simulink model "DoubleTankSim_FeedbackLin"  (R2025b)
settings: Solver=ode5  StartTime=0.0  StopTime=1500  FixedStep=Ts  RelTol=1e-3  EnableMultiTasking=on
values from neighbouring files (symbols this model uses):
  a_1 = 0.15025    [LabC.m]
  a_2 = 0.15615    [LabC.m]
  At = 33    [LabC.m]
  g = 981    [LabC.m]
  h_0 = 3.2    [LabC.m]
  h_1 = [2.5 3 3.5 4 4.5 5 5.5 6 6.5 7 7.5 8 8.5 9 9.5 10 10.5 11 11.5 12 12.5 13 13.5 14.5 15]    [LabC.m]
  h_2 = [3 3.5 4 4.5 5 5.5 6 6.5 7 7.5 8 8.5 9 9.5 10 10.5 11 11.5 12 12.5 13 13.5 14 14.5 15]    [LabC.m]
  h_2_V = [0.75 1.03 1.47 1.85 2.22 2.61 2.93 3.35 3.72 4.09 4.49 4.88 5.21 5.62 6.00 6.33 6.75  7.13 7.50 7.94 8.29 8.65 9.03 9.38 9.77]    [LabC.m]
  height_limit = 15.5    [LabC.m]
  height_safe = 0.9 * height_limit    (= 13.95)    [LabC.m]
  Kd = 12 * zeta * omega_n    (= 0.64)    [LabC.m]
  Ki = 10 * zeta * omega_n^3    (= 0.00151703703704)    [LabC.m]
  Kp = omega_n^2 * (1 + 20*zeta^2)    (= 0.0597333333333)    [LabC.m]
  N = 1    [LabC.m]
  omega_n = 4/(zeta*T_s_cl)    (= 0.0533333333333)    [LabC.m]
  Q = [variance 0 0 ... (first row only)    [LabC.m]
  R = 1    [LabC.m]
  R_2d = diag([1, 1])    [LabC.m]
  tau = T_s_cl/2    (= 37.5)    [LabC.m]
  Ts = 0.02    [LabC.m]
undefined symbols (not defined in the file or in its folder): h_1_V, National_Instruments, PCIe
libraries: sldrtlib x2, simulink x2, slpidlib x2
settings Model: Creator=William  LastModifiedBy=William
settings SolverCC: AutoInsertRateTranBlk=on

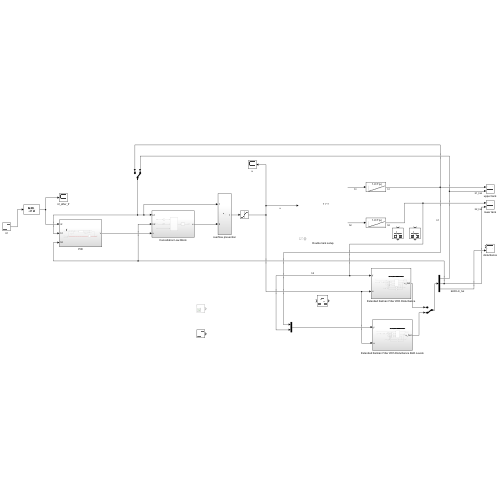
[thumbnail: Simulink's stored preview of the top-level diagram]
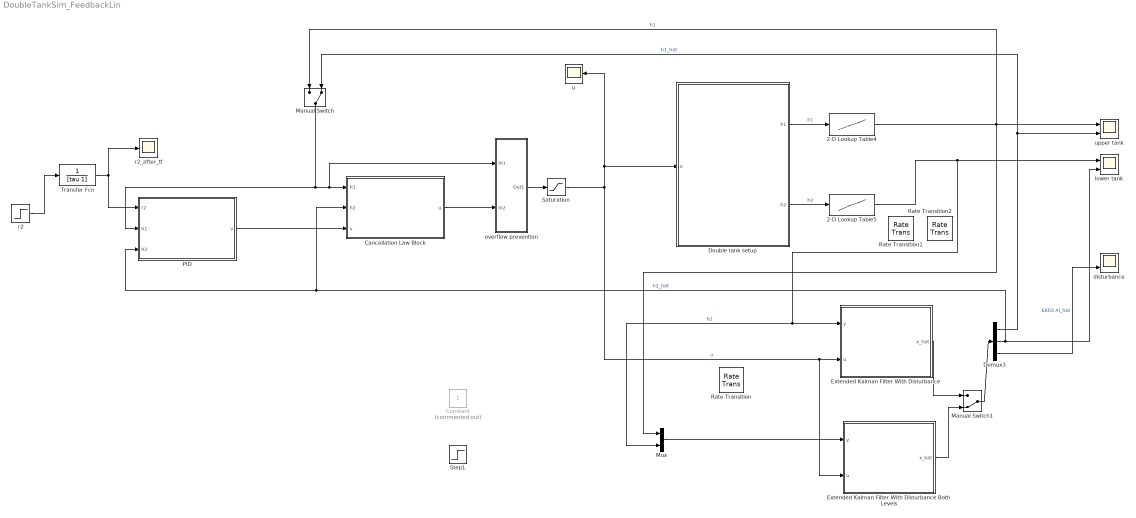
== system DoubleTankSim_FeedbackLin ==
  2-D Lookup Table4 : Lookup_n-D  NumberOfTableDimensions=1  BreakpointsForDimension1=x  BreakpointsForDimension2=[1:3]  Table=y  RndMeth=Simplest  mask{x=h_1_V, y=h_1}
      mask prompts: x "Values on x-axis"; y "Values on y-axis"
  2-D Lookup Table5 : Lookup_n-D  NumberOfTableDimensions=1  BreakpointsForDimension1=x  BreakpointsForDimension2=[1:3]  Table=y  RndMeth=Simplest  mask{x=h_2_V, y=h_2}
      mask prompts: x "Values on x-axis"; y "Values on y-axis"
  Cancellation Law Block : Subsystem
  Constant : Constant  Commented=on
  Demux3 : Demux  Outputs=3
  Double tank setup : Subsystem  AncestorBlock=R7014E_lib/Double tank setup  StopFcn=|  mask(Realtime interface for the tank process){ts=0.02, h1_ch=0, h2_ch=1, u_ch=0}
      | chn =get_param(gcb,'u_ch');                          
      | s = daq.createSession('ni');                         
      | channel = ['ao',chn];                                
      | s.addAnalogOutputChannel('Dev1', channel, 'Voltage');
      | x = zeros(5,1);                                      
      | s.queueOutputData(x);                                
      | lh = s.addlistener('DataRequired', ...               
      | @(src,event) src.queueOutputData(x));                
      | s.startBackground();                                 
      | s.wait();                                            
      | s.stop();                                            
      | delete(lh);                                          
      | clear chn;                                           
      | clear s;                                             
      | clear channel;                                       
      | clear lh;                                            
      | clear x;
      mask prompts: ts "Sample time"; h1_ch "A/D Channel for upper tank"; h2_ch "A/D Channel for lower tank"; u_ch "D/A Channel for pump"
      mask help:
      | This block represents the physical interface from the computer to the tank process.
      |
      | The input u is the voltage that is provided for the pump, the output h1 is the measured level in the upper tank in [V] and the output h2 is the
      | measured level in the lower tank in [V].
      |
      | You need to provide the sample rate at which the voltage to the pump is updated and the level measurements are sampled. The sample rate should not be less than 0.02 seconds.
      mask Display:
      | x=363;
      | y=381;
      | image(imread('tank_icon.jpg'));
      | text(250/x,309/y,'Sensor');
      | text(260/x,169/y,'Sensor');
      | text(335/x,289/y,'A');
      | text(351/x,283/y,'D');
      | text(335/x,100/y,'A');
      | text(351/x,95/y,'D');
      | text(22/x,187/y,'A');
      | text(5/x,195/y,'D');
      | text(225/x,278/y,'h_1','texmode','on');
      | text(225/x,146/y,'h_2','texmode','on');
      | text(300/x,270/y,sprintf('AI-%d',h1_ch));
      | text(300/x,80/y,sprintf('AI-%d',h2_ch));
      | text(40/x,173/y,sprintf('AO-%d',u_ch));
  Extended Kalman Filter With Disturbance : Subsystem
  Extended Kalman Filter With Disturbance Both Levels : Subsystem
  Manual Switch : ManualSwitch  CurrentSetting=0
  Manual Switch1 : ManualSwitch  CurrentSetting=0
  Mux : Mux  Inputs=2
  PID : Subsystem
  Rate Transition : RateTransition  OutPortSampleTime=Ts
  Rate Transition1 : RateTransition  OutPortSampleTime=Ts
  Rate Transition2 : RateTransition  OutPortSampleTime=Ts
  Saturation : Saturate  UpperLimit=10  LowerLimit=0
  Step1 : Step  Time=750  Before=1  After=1.25  SampleTime=0
  Transfer Fcn : TransferFcn  Denominator=[tau 1]
  disturbance : Scope  NumInputPorts=2
      settings: ActiveDisplayYMinimum=-0.015496470014474377  ActiveDisplayYMaximum=0.13931374108372324  DataLoggingVariableName=ScopeData2
  lower tank : Scope  NumInputPorts=2
      settings: ActiveDisplayYMinimum=-1.8057811743118082  ActiveDisplayYMaximum=15.777371038796296
  overflow prevention : Subsystem
  r2 : Step  Time=500  Before=8  After=13.95  SampleTime=0
  r2_after_tf : Scope
      settings: ActiveDisplayYMinimum=-1.7437499999996442  ActiveDisplayYMaximum=15.693749999996802  DataLoggingVariableName=ScopeData4
  u : Scope
      settings: ActiveDisplayYMinimum=-1.2499999999999998  ActiveDisplayYMaximum=11.25  DataLoggingVariableName=ScopeData3
  upper tank : Scope  NumInputPorts=2
      settings: ActiveDisplayYMinimum=-1.9029859274386325  ActiveDisplayYMaximum=16.774636482282123
  wires:
  overflow prevention/1(Out1) -> Saturation/1
  Mux/1 -> Extended Kalman Filter With Disturbance Both Levels/1(y)
  Extended Kalman Filter With Disturbance Both Levels/1(x_hat) -> Manual Switch1/2
  Manual Switch1/1 -> Demux3/1
  PID/1(v) -> Cancellation Law Block/3(v)
  r2/1 -> Transfer Fcn/1
  Manual Switch/1 -> PID/2(h1), overflow prevention/1(In1), Cancellation Law Block/1(h1)
  Transfer Fcn/1 -> r2_after_tf/1, PID/1(r2)
  Extended Kalman Filter With Disturbance/1(x_hat) -> Manual Switch1/1
  Demux3/3 -> disturbance/2  "EKFD Al_hat"
  Cancellation Law Block/1(u) -> overflow prevention/2(In2)
  Saturation/1 -> Extended Kalman Filter With Disturbance Both Levels/2(u), Extended Kalman Filter With Disturbance/2(u), u/1, Double tank setup/1(u)  "u"
  Demux3/1 -> upper tank/2, Manual Switch/2  "h1_hat"
  Double tank setup/1(h1) -> 2-D Lookup Table4/1  "h1"
  Demux3/2 -> PID/3(h2), Cancellation Law Block/2(h2), lower tank/2  "h2_hat"
  Double tank setup/2(h2) -> 2-D Lookup Table5/1  "h2"
  2-D Lookup Table4/1 -> Mux/1, upper tank/1, Manual Switch/1  "h1"
  2-D Lookup Table5/1 -> Mux/2, Extended Kalman Filter With Disturbance/1(y), lower tank/1  "h2"

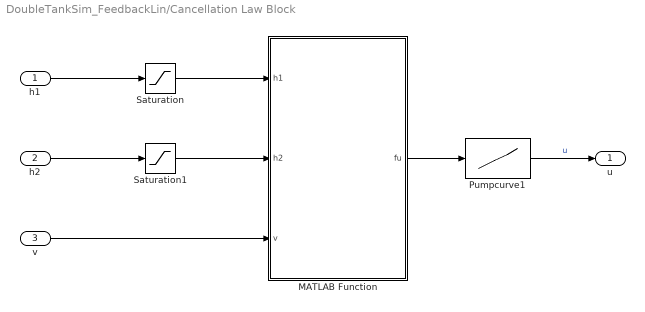
== system DoubleTankSim_FeedbackLin/Cancellation Law Block ==
  h1 : Inport
  h2 : Inport  Port=2
  v : Inport  Port=3
  MATLAB Function : MATLAB Function  TreatAsAtomicUnit=on
  Pumpcurve1 : Lookup_n-D  NumberOfTableDimensions=1  BreakpointsForDimension1=x  BreakpointsForDimension2=[1:3]  Table=y  RndMeth=Simplest  mask{x=[16.47,20.75,24.52,27.63,30.06,32.49,34.80,40.28,48.24,52.43], y=[0.5,1,1.5,2,2.5,3,3.5,5,8,10]}
      mask prompts: x "Values on x-axis"; y "Values on y-axis"
  Saturation : Saturate  UpperLimit=15.5  LowerLimit=0.001
  Saturation1 : Saturate  UpperLimit=15.5  LowerLimit=0.001
  u : Outport
  wires:
  MATLAB Function/1(fu) -> Pumpcurve1/1
  h1/1 -> Saturation/1
  h2/1 -> Saturation1/1
  Pumpcurve1/1 -> u/1  "u"
  v/1 -> MATLAB Function/3(v)
  Saturation/1 -> MATLAB Function/1(h1)
  Saturation1/1 -> MATLAB Function/2(h2)

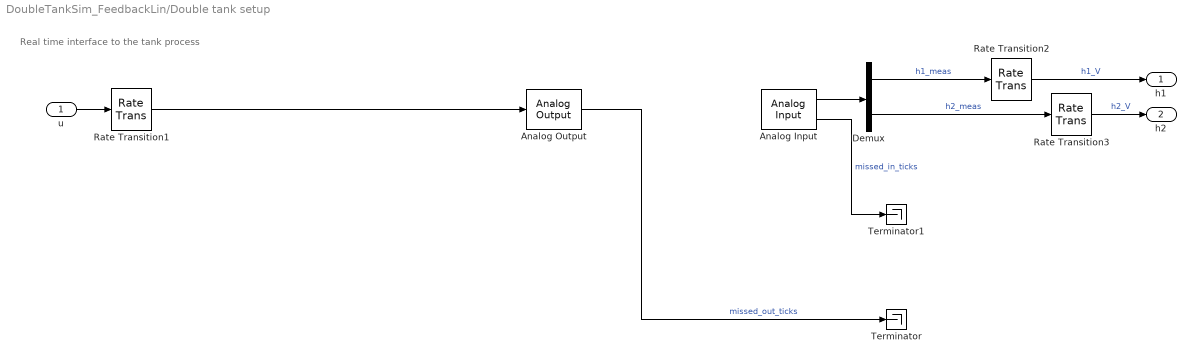
== system DoubleTankSim_FeedbackLin/Double tank setup ==
  note: Real time interface to the tank process
  u : Inport
  Analog Input : sldrtlib/Analog Input  SampleTime=ts  MaxMissedTicks=500000000  ShowMissedTicks=on  YieldWhenWaiting=off  DrvName=National_Instruments/PCIe-6321  DrvAddress=4294967295  DrvOptions=[0 0 0 0 0 0 0]  Channels=[h1_ch+1,h2_ch+1]  RangeMode=1  VoltRange=1  DataType=1
      settings: AttributesFormatString=National Instruments\nPCIe-6321 [auto]
  Analog Output : sldrtlib/Analog Output  SampleTime=ts  MaxMissedTicks=500000000  ShowMissedTicks=on  YieldWhenWaiting=off  DrvName=National_Instruments/PCIe-6321  DrvAddress=4294967295  DrvOptions=[0 0 0 0 0 0 0]  Channels=u_ch+1  RangeMode=1  VoltRange=1  InitialValue=0  FinalValue=0
      settings: AttributesFormatString=National Instruments\nPCIe-6321 [auto]
  Demux : Demux  Outputs=2
  Rate Transition1 : RateTransition  OutPortSampleTime=ts
  Rate Transition2 : RateTransition
  Rate Transition3 : RateTransition
  Terminator : Terminator
  Terminator1 : Terminator
  h1 : Outport
  h2 : Outport  Port=2
  wires:
  u/1 -> Rate Transition1/1
  Analog Output/1 -> Terminator/1  "missed_out_ticks"
  Analog Input/1 -> Demux/1
  Demux/1 -> Rate Transition2/1  "h1_meas"
  Demux/2 -> Rate Transition3/1  "h2_meas"
  Analog Input/2 -> Terminator1/1  "missed_in_ticks"
  Rate Transition2/1 -> h1/1  "h1_V"
  Rate Transition3/1 -> h2/1  "h2_V"
  Rate Transition1/1 -> Analog Output/1

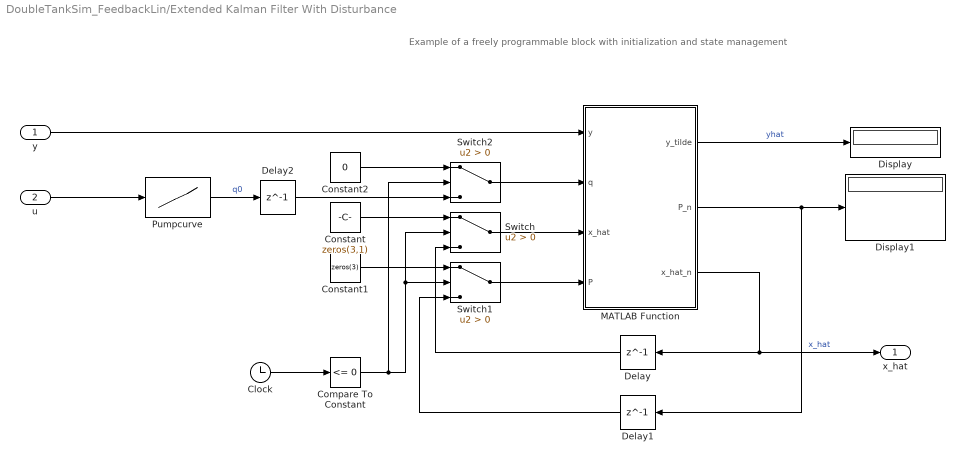
== system DoubleTankSim_FeedbackLin/Extended Kalman Filter With Disturbance ==
  note: Example of a freely programmable block with initialization and state management
  y : Inport
  u : Inport  Port=2
  Clock : Clock
  Compare To Constant : simulink/Logic and Bit Operations/Compare To Constant  relop=<=  const=0  OutDataTypeStr=boolean
  Constant : Constant  Value=zeros(3,1)
  Constant1 : Constant  Value=zeros(3)
  Constant2 : Constant  Value=0
  Delay : Delay  DelayLength=1  InitialCondition=0
  Delay1 : Delay  DelayLength=1  InitialCondition=0
  Delay2 : Delay  DelayLength=1  InitialCondition=0
  Display : Display
  Display1 : Display
  MATLAB Function : MATLAB Function  TreatAsAtomicUnit=on
  Pumpcurve : Lookup_n-D  NumberOfTableDimensions=1  BreakpointsForDimension1=x  BreakpointsForDimension2=[1:3]  Table=y  RndMeth=Simplest  mask{x=[0.5,1,1.5,2,2.5,3,3.5,5,8,10], y=[16.47,20.75,24.52,27.63,30.06,32.49,34.80,40.28,48.24,52.43]}
      mask prompts: x "Values on x-axis"; y "Values on y-axis"
  Switch : Switch  Criteria=u2 > Threshold  SaturateOnIntegerOverflow=off  InputSameDT=off
  Switch1 : Switch  Criteria=u2 > Threshold  SaturateOnIntegerOverflow=off  InputSameDT=off
  Switch2 : Switch  Criteria=u2 > Threshold  SaturateOnIntegerOverflow=off  InputSameDT=off
  x_hat : Outport  PortDimensions=3
  wires:
  Delay/1 -> Switch/3
  Switch/1 -> MATLAB Function/3(x_hat)
  Constant1/1 -> Switch1/1
  Compare To Constant/1 -> Switch2/2, Switch/2, Switch1/2
  Constant/1 -> Switch/1
  MATLAB Function/1(y_tilde) -> Display/1  "yhat"
  MATLAB Function/2(P_n) -> Delay1/1, Display1/1
  Clock/1 -> Compare To Constant/1
  Switch1/1 -> MATLAB Function/4(P)
  y/1 -> MATLAB Function/1(y)
  Delay1/1 -> Switch1/3
  Switch2/1 -> MATLAB Function/2(q)
  Constant2/1 -> Switch2/1
  Delay2/1 -> Switch2/3
  Pumpcurve/1 -> Delay2/1  "q0"
  u/1 -> Pumpcurve/1
  MATLAB Function/3(x_hat_n) -> Delay/1, x_hat/1  "x_hat"

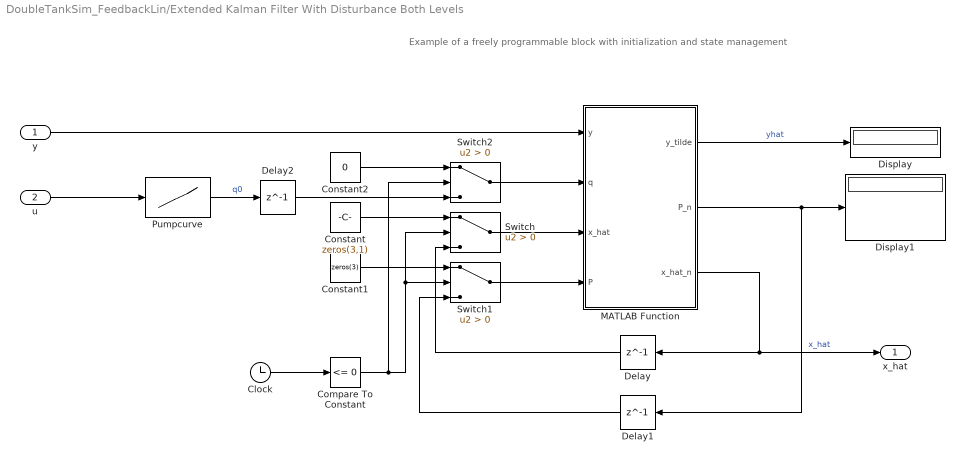
== system DoubleTankSim_FeedbackLin/Extended Kalman Filter With Disturbance Both Levels ==
  note: Example of a freely programmable block with initialization and state management
  y : Inport
  u : Inport  Port=2
  Clock : Clock
  Compare To Constant : simulink/Logic and Bit Operations/Compare To Constant  relop=<=  const=0  OutDataTypeStr=boolean
  Constant : Constant  Value=zeros(3,1)
  Constant1 : Constant  Value=zeros(3)
  Constant2 : Constant  Value=0
  Delay : Delay  DelayLength=1  InitialCondition=0
  Delay1 : Delay  DelayLength=1  InitialCondition=0
  Delay2 : Delay  DelayLength=1  InitialCondition=0
  Display : Display
  Display1 : Display
  MATLAB Function : MATLAB Function  TreatAsAtomicUnit=on
  Pumpcurve : Lookup_n-D  NumberOfTableDimensions=1  BreakpointsForDimension1=x  BreakpointsForDimension2=[1:3]  Table=y  RndMeth=Simplest  mask{x=[0.5,1,1.5,2,2.5,3,3.5,5,8,10], y=[16.47,20.75,24.52,27.63,30.06,32.49,34.80,40.28,48.24,52.43]}
      mask prompts: x "Values on x-axis"; y "Values on y-axis"
  Switch : Switch  Criteria=u2 > Threshold  SaturateOnIntegerOverflow=off  InputSameDT=off
  Switch1 : Switch  Criteria=u2 > Threshold  SaturateOnIntegerOverflow=off  InputSameDT=off
  Switch2 : Switch  Criteria=u2 > Threshold  SaturateOnIntegerOverflow=off  InputSameDT=off
  x_hat : Outport  PortDimensions=3
  wires:
  Delay/1 -> Switch/3
  Switch/1 -> MATLAB Function/3(x_hat)
  Constant1/1 -> Switch1/1
  Compare To Constant/1 -> Switch2/2, Switch/2, Switch1/2
  Constant/1 -> Switch/1
  MATLAB Function/1(y_tilde) -> Display/1  "yhat"
  MATLAB Function/2(P_n) -> Delay1/1, Display1/1
  Clock/1 -> Compare To Constant/1
  Switch1/1 -> MATLAB Function/4(P)
  y/1 -> MATLAB Function/1(y)
  Delay1/1 -> Switch1/3
  Switch2/1 -> MATLAB Function/2(q)
  Constant2/1 -> Switch2/1
  Delay2/1 -> Switch2/3
  Pumpcurve/1 -> Delay2/1  "q0"
  u/1 -> Pumpcurve/1
  MATLAB Function/3(x_hat_n) -> Delay/1, x_hat/1  "x_hat"

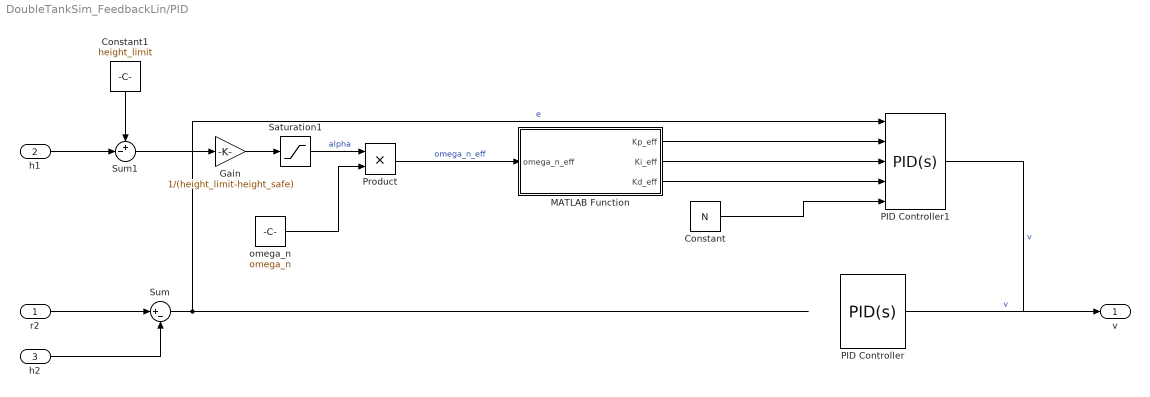
== system DoubleTankSim_FeedbackLin/PID ==
  r2 : Inport
  h1 : Inport  Port=2
  h2 : Inport  Port=3
  Constant : Constant  Value=N
  Constant1 : Constant  Value=height_limit
  Gain : Gain  Gain=1/(height_limit-height_safe)
  MATLAB Function : MATLAB Function  TreatAsAtomicUnit=on
  PID Controller : slpidlib/PID Controller  Controller=PID  Form=Parallel  TimeDomain=Continuous-time  UseExternalTs=off  SampleTime=-1  IntegratorMethod=Forward Euler  FilterMethod=Forward Euler  ControllerParametersSource=internal  P=Kp  I=Ki  UseKiTs=off  D=Kd  UseExternalDerivativeSource=off  N=N  UseFilter=on  TunerSelectOption=Transfer Function Based (PID Tuner App)  InitialConditionSource=internal  InitialConditionForIntegrator=0  InitialConditionForFilter=0  DifferentiatorICPrevScaledInput=0  ExternalReset=none  TrackingMode=off  Kt=1  LimitOutput=off  SatLimitsSource=internal  UpperSaturationLimit=10  LowerSaturationLimit=0  LinearizeAsGain=on  AntiWindupMode=back-calculation  Kb=1/Kd  LimitIntegrator=off  UpperIntegratorSaturationLimit=inf  LowerIntegratorSaturationLimit=-inf  POutMin=[]  POutMax=[]  IOutMin=[]  IOutMax=[]  DOutMin=[]  DOutMax=[]  NOutMin=[]  NOutMax=[]  SumOutMin=[]  SumOutMax=[]  SaturationOutMin=[]  SaturationOutMax=[]  PParamMin=[]  PParamMax=[]  IParamMin=[]  IParamMax=[]  DParamMin=[]  DParamMax=[]  NParamMin=[]  NParamMax=[]  KbParamMin=[]  KbParamMax=[]  KtParamMin=[]  KtParamMax=[]  KbOutMin=[]  KbOutMax=[]  KtOutMin=[]  KtOutMax=[]  IntegratorOutMin=[]  IntegratorOutMax=[]  FilterOutMin=[]  FilterOutMax=[]  SumI1OutMin=[]  SumI1OutMax=[]  SumI2OutMin=[]  SumI2OutMax=[]  SumI3OutMin=[]  SumI3OutMax=[]  SumI4OutMin=[]  SumI4OutMax=[]  SumDOutMin=[]  SumDOutMax=[]  DifferentiatorOutMin=[]  DifferentiatorOutMax=[]  FilterDiffOutCoefMin=[]  FilterDiffOutCoefMax=[]  ReciprocalOutMin=[]  ReciprocalOutMax=[]  SumDenOutMin=[]  SumDenOutMax=[]  SumNumOutMin=[]  SumNumOutMax=[]  DivideOutMin=[]  DivideOutMax=[]  UdiffTsProdOutMin=[]  UdiffTsProdOutMax=[]  NTsProdOutMin=[]  NTsProdOutMax=[]  UintegralTsProdOutMin=[]  UintegralTsProdOutMax=[]  UngainTsProdOutMin=[]  UngainTsProdOutMax=[]  ClampingZeroOutDataTypeStr=Inherit: Inherit via back propagation  ClampingZeroOutMin=[]  ClampingZeroOutMax=[]  FilterDenConstantOutDataTypeStr=Inherit: Inherit via back propagation  FilterDenConstantOutMin=[]  FilterDenConstantOutMax=[]  PCopyOutDataTypeStr=Inherit: Inherit via back propagation  PCopyOutMin=[]  PCopyOutMax=[]  NCopyOutDataTypeStr=Inherit: Inherit via back propagation  NCopyOutMin=[]  NCopyOutMax=[]  IntegratorContinuousStateAttributes=''  IntegratorStateMustResolveToSignalObject=off  IntegratorRTWStateStorageClass=Auto  FilterContinuousStateAttributes=''  FilterStateMustResolveToSignalObject=off  FilterRTWStateStorageClass=Auto  ParallelPVariant=InternalParameters  IdealPVariant=Disabled  IVariant=InternalParameters  DVariant=InternalParameters  IntegratorVariant=Continuous  SatVariant=Disabled  AWVariant=Passthrough  PCopyVariant=Disabled  TRVariant=Disabled  FdbkBlocksVariant=Forward  IdealPFdbkVariant=Disabled  SatFdbkVariant=Disabled  DerivativeFilterVariant=ContFilter  NVariant=InternalParameters  NCopyVariant=Disabled  FilterICVariant=InternalICsFilter  IntegratorICVariant=InternalICs  ExternalResetVariant=Disabled  TRSumVariant=Passthrough  SumFdbkVariant=Disabled  SumVariant=Sum_PID  TsampFilterVariant=InternalTs  TsampNgainVariant=Passthrough  TsampIntegralVariant=Disabled_SignalSpec  ExternalSaturationOutDataTypeStr=Inherit: Same as second input  DerivativeSourceVariant=ErrorSignal  PreIntVariant=InternalPreInt
  PID Controller1 : slpidlib/PID Controller  Controller=PID  Form=Parallel  TimeDomain=Continuous-time  UseExternalTs=off  SampleTime=-1  IntegratorMethod=Forward Euler  FilterMethod=Forward Euler  ControllerParametersSource=external  P=Kp  I=Ki  UseKiTs=off  D=Kd  UseExternalDerivativeSource=off  N=1  UseFilter=on  TunerSelectOption=Transfer Function Based (PID Tuner App)  InitialConditionSource=internal  InitialConditionForIntegrator=0  InitialConditionForFilter=0  DifferentiatorICPrevScaledInput=0  ExternalReset=none  TrackingMode=off  Kt=1  LimitOutput=off  SatLimitsSource=internal  UpperSaturationLimit=10  LowerSaturationLimit=0  LinearizeAsGain=on  AntiWindupMode=back-calculation  Kb=1/Kd  LimitIntegrator=off  UpperIntegratorSaturationLimit=inf  LowerIntegratorSaturationLimit=-inf  POutMin=[]  POutMax=[]  IOutMin=[]  IOutMax=[]  DOutMin=[]  DOutMax=[]  NOutMin=[]  NOutMax=[]  SumOutMin=[]  SumOutMax=[]  SaturationOutMin=[]  SaturationOutMax=[]  PParamMin=[]  PParamMax=[]  IParamMin=[]  IParamMax=[]  DParamMin=[]  DParamMax=[]  NParamMin=[]  NParamMax=[]  KbParamMin=[]  KbParamMax=[]  KtParamMin=[]  KtParamMax=[]  KbOutMin=[]  KbOutMax=[]  KtOutMin=[]  KtOutMax=[]  IntegratorOutMin=[]  IntegratorOutMax=[]  FilterOutMin=[]  FilterOutMax=[]  SumI1OutMin=[]  SumI1OutMax=[]  SumI2OutMin=[]  SumI2OutMax=[]  SumI3OutMin=[]  SumI3OutMax=[]  SumI4OutMin=[]  SumI4OutMax=[]  SumDOutMin=[]  SumDOutMax=[]  DifferentiatorOutMin=[]  DifferentiatorOutMax=[]  FilterDiffOutCoefMin=[]  FilterDiffOutCoefMax=[]  ReciprocalOutMin=[]  ReciprocalOutMax=[]  SumDenOutMin=[]  SumDenOutMax=[]  SumNumOutMin=[]  SumNumOutMax=[]  DivideOutMin=[]  DivideOutMax=[]  UdiffTsProdOutMin=[]  UdiffTsProdOutMax=[]  NTsProdOutMin=[]  NTsProdOutMax=[]  UintegralTsProdOutMin=[]  UintegralTsProdOutMax=[]  UngainTsProdOutMin=[]  UngainTsProdOutMax=[]  ClampingZeroOutDataTypeStr=Inherit: Inherit via back propagation  ClampingZeroOutMin=[]  ClampingZeroOutMax=[]  FilterDenConstantOutDataTypeStr=Inherit: Inherit via back propagation  FilterDenConstantOutMin=[]  FilterDenConstantOutMax=[]  PCopyOutDataTypeStr=Inherit: Inherit via back propagation  PCopyOutMin=[]  PCopyOutMax=[]  NCopyOutDataTypeStr=Inherit: Inherit via back propagation  NCopyOutMin=[]  NCopyOutMax=[]  IntegratorContinuousStateAttributes=''  IntegratorStateMustResolveToSignalObject=off  IntegratorRTWStateStorageClass=Auto  FilterContinuousStateAttributes=''  FilterStateMustResolveToSignalObject=off  FilterRTWStateStorageClass=Auto  ParallelPVariant=ExternalParameters  IdealPVariant=Disabled  IVariant=ExternalParameters  DVariant=ExternalParameters  IntegratorVariant=Continuous  SatVariant=Disabled  AWVariant=Passthrough  PCopyVariant=Disabled  TRVariant=Disabled  FdbkBlocksVariant=Forward  IdealPFdbkVariant=Disabled  SatFdbkVariant=Disabled  DerivativeFilterVariant=ContFilter  NVariant=ExternalParameters  NCopyVariant=Disabled  FilterICVariant=InternalICsFilter  IntegratorICVariant=InternalICs  ExternalResetVariant=Disabled  TRSumVariant=Passthrough  SumFdbkVariant=Disabled  SumVariant=Sum_PID  TsampFilterVariant=InternalTs  TsampNgainVariant=Passthrough  TsampIntegralVariant=Disabled_SignalSpec  ExternalSaturationOutDataTypeStr=Inherit: Same as second input  DerivativeSourceVariant=ErrorSignal  PreIntVariant=InternalPreInt
  Product : Product
  Saturation1 : Saturate  UpperLimit=1  LowerLimit=0
  Sum : Sum  Inputs=|+-
  Sum1 : Sum  Inputs=+-|
  omega_n : Constant  Value=omega_n
  v : Outport
  wires:
  h2/1 -> Sum/2
  Sum/1 -> PID Controller1/1  "e"
  PID Controller/1 -> ?  "v"
  r2/1 -> Sum/1
  h1/1 -> Sum1/2
  Sum1/1 -> Gain/1
  Product/1 -> MATLAB Function/1(omega_n_eff)  "omega_n_eff"
  Constant1/1 -> Sum1/1
  Saturation1/1 -> Product/1  "alpha"
  Gain/1 -> Saturation1/1
  omega_n/1 -> Product/2
  MATLAB Function/1(Kp_eff) -> PID Controller1/2
  MATLAB Function/2(Ki_eff) -> PID Controller1/3
  MATLAB Function/3(Kd_eff) -> PID Controller1/4
  Constant/1 -> PID Controller1/5
  PID Controller1/1 -> v/1  "v"

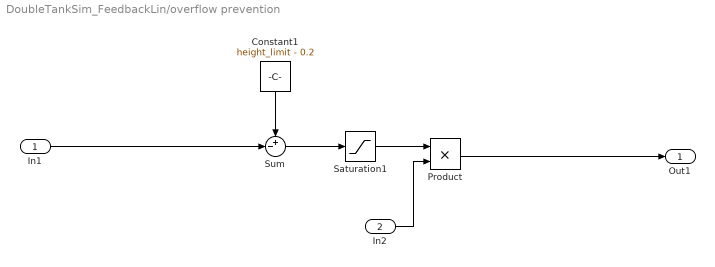
== system DoubleTankSim_FeedbackLin/overflow prevention ==
  In1 : Inport
  In2 : Inport  Port=2
  Constant1 : Constant  Value=height_limit - 0.2
  Product : Product
  Saturation1 : Saturate  UpperLimit=1  LowerLimit=0
  Sum : Sum  Inputs=+-|
  Out1 : Outport
  wires:
  Constant1/1 -> Sum/1
  Product/1 -> Out1/1
  Saturation1/1 -> Product/1
  Sum/1 -> Saturation1/1
  In2/1 -> Product/2
  In1/1 -> Sum/2

== matlab function DoubleTankSim_FeedbackLin/Extended Kalman Filter With Disturbance Both Levels/MATLAB Function ==
  data: y input; q input; x_hat input; At parameter; a_1 parameter; a_2 parameter; h_0 parameter; y_tilde output; P input; P_n output; x_hat_n output; Q parameter; R_2d parameter; g parameter; Ts parameter
function [y_tilde, P_n, x_hat_n] = fcn(y, q, x_hat, At, a_1, a_2, h_0, P, Q, R_2d, g, Ts)

% Linearization
h_hat1 = x_hat(1);
h_hat2 = x_hat(2);
a_l = x_hat(3);

sqrt1 = sqrt(2*g*(max([h_hat1+h_0,0])));
sqrt2 = sqrt(2*g*(max([h_hat2+h_0,0])));

A = [-(a_1 + a_l)*g/At/sqrt1, 0,              -sqrt1/At;
     a_1*g/At/sqrt1,           -a_2*g/At/sqrt2, 0
     0,                       0,              0];

C = [1 0 0;
    0 1 0];

Ad = eye(size(A)) + Ts * A;

% Predict
x_hat_dot = [(q - (a_1 + a_l)*sqrt1)/At; 
             (a_1*sqrt1 - a_2*sqrt2)/At;
             0];
x_hat_n = x_hat + x_hat_dot .* Ts;
P_n = Ad * P * Ad' + Q;

% Update
y_tilde = y - C * x_hat_n;
S = C * P_n * C' + R_2d;
K = P_n * C' * inv(S);
x_hat_n = x_hat_n + K * y_tilde;
P_n = (eye(size(A)) - K * C) * P_n;   
y_tilde = y - C * x_hat_n;

== matlab function DoubleTankSim_FeedbackLin/Cancellation Law Block/MATLAB Function ==
  data: h1 input; fu output; h2 input; v input; h_0 parameter; At parameter; a_1 parameter; a_2 parameter; g parameter
function fu = fcn(h1, h2, v, h_0, At, a_1, a_2, g)

% this function computes f(u) so that all the non-linear terms are canceled

q1 = sqrt(2*g*(h1 + h_0));  % ← Math Function block (sqrt), with Gain 2*g beforehand
q2 = sqrt(2*g*(h2 + h_0));  % ← same structure

phi = -(a_1^2*g/At^2) - (a_2*g*(a_1*q1 - a_2*q2))/(At^2*q2);

beta = (a_1*g) / (At^2*q1);

fu = (v - phi) / beta;

== matlab function DoubleTankSim_FeedbackLin/PID/MATLAB Function ==
  data: omega_n_eff input; Kp_eff output; Ki_eff output; Kd_eff output; zeta parameter
function [Kp_eff, Ki_eff, Kd_eff] = fcn(omega_n_eff, zeta)

Kp_eff = omega_n_eff^2 * (1 + 20*zeta^2);
Ki_eff = 10 * zeta * omega_n_eff^3;
Kd_eff = 12 * zeta * omega_n_eff;

== matlab function DoubleTankSim_FeedbackLin/Extended Kalman Filter With Disturbance/MATLAB Function ==
  data: y input; q input; x_hat input; At parameter; a_1 parameter; a_2 parameter; h_0 parameter; y_tilde output; P input; P_n output; x_hat_n output; Q parameter; R parameter; g parameter; Ts parameter
function [y_tilde, P_n, x_hat_n] = fcn(y, q, x_hat, At, a_1, a_2, h_0, P, Q, R, g, Ts)

% Linearization
h_hat1 = x_hat(1);
h_hat2 = x_hat(2);
a_l = x_hat(3);

sqrt1 = sqrt(2*g*(max([h_hat1+h_0,0])));
sqrt2 = sqrt(2*g*(max([h_hat2+h_0,0])));

A = [-(a_1 + a_l)*g/At/sqrt1, 0,              -sqrt1/At;
     a_1*g/At/sqrt1,           -a_2*g/At/sqrt2, 0
     0,                       0,              0];

C = [0 1 0];

Ad = eye(size(A)) + Ts * A;

% Predict
x_hat_dot = [(q - (a_1 + a_l)*sqrt1)/At; 
             (a_1*sqrt1 - a_2*sqrt2)/At;
             0];
x_hat_n = x_hat + x_hat_dot .* Ts;
P_n = Ad * P * Ad' + Q;

% Update
y_tilde = y - C * x_hat_n;
S = C * P_n * C' + R;
K = P_n * C' * inv(S);
x_hat_n = x_hat_n + K * y_tilde;
P_n = (eye(size(A)) - K * C) * P_n;   
y_tilde = y - C * x_hat_n;
